simulink model "topic1——5"  (R2019b)
settings: Solver=VariableStepAuto  StartTime=0.0  StopTime=0.12  RelTol=1e-3
libraries: powerlib x14, powerlib_meascontrol x7
settings Model: Creator=96547  LastModifiedBy=96547

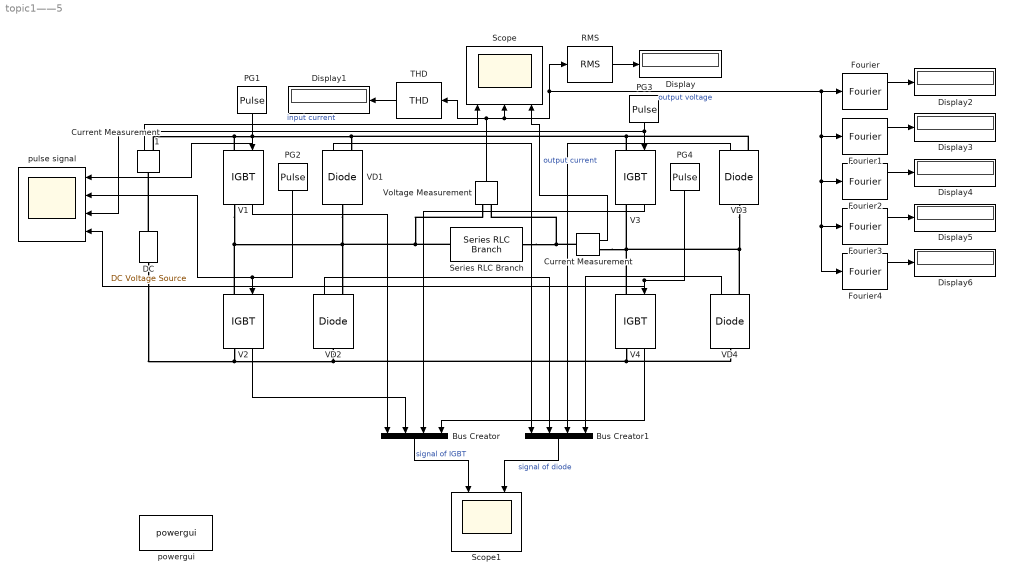
== system topic1——5 ==
  Bus Creator : BusCreator  Inputs=4
  Bus Creator1 : BusCreator  Inputs=4
  Current Measurement : powerlib/Measurements/Current Measurement  PhasorSimulation=off  OutputType=Complex  PSBequivalent=0
      settings: SourceProductName=Simscape Electrical
  Current Measurement1 : powerlib/Measurements/Current Measurement  PhasorSimulation=off  OutputType=Complex  PSBequivalent=0
      settings: SourceProductName=Simscape Electrical
  DC : powerlib/Electrical Sources/DC Voltage Source  Amplitude=400  Measurements=None
      settings: SourceProductName=Simscape Electrical
  Display{,1..6} (7 alike) : Display
  Fourier : powerlib_meascontrol/Measurements/Fourier  Freq=50  n=3  InInit=[0, 0]  Ts=0
      settings: SourceProductName=Simscape Electrical
  Fourier1 : powerlib_meascontrol/Measurements/Fourier  Freq=60  n=1  InInit=[0, 0]  Ts=0
      settings: SourceProductName=Simscape Electrical
  Fourier2 : powerlib_meascontrol/Measurements/Fourier  Freq=50  n=5  InInit=[0, 0]  Ts=0
      settings: SourceProductName=Simscape Electrical
  Fourier3 : powerlib_meascontrol/Measurements/Fourier  Freq=50  n=7  InInit=[0, 0]  Ts=0
      settings: SourceProductName=Simscape Electrical
  Fourier4 : powerlib_meascontrol/Measurements/Fourier  Freq=50  n=9  InInit=[0, 0]  Ts=0
      settings: SourceProductName=Simscape Electrical
  PG1 : DiscretePulseGenerator  PulseType=Time based  Period=0.02  PulseWidth=50
  PG2 : DiscretePulseGenerator  PulseType=Time based  Period=0.02  PulseWidth=50  PhaseDelay=0.01
  PG3 : DiscretePulseGenerator  PulseType=Time based  Period=0.02  PulseWidth=50  PhaseDelay=0.02*(1/6)
  PG4 : DiscretePulseGenerator  PulseType=Time based  Period=0.02  PulseWidth=50  PhaseDelay=0.01+0.02*(1/6)
  RMS : powerlib_meascontrol/Measurements/RMS  TrueRMS=on  Freq=60  RMSInit=120  Ts=0
      settings: SourceProductName=Simscape Electrical
  Scope : Scope  NumInputPorts=3
  Scope1 : Scope  NumInputPorts=2
  Series RLC Branch : powerlib/Elements/Series RLC Branch  LConnTagsString=__new0  RConnTagsString=__new0  BranchType=R  Resistance=8  Inductance=1e-3  SetiL0=off  InitialCurrent=0  Capacitance=1e-6  Setx0=off  InitialVoltage=0  Measurements=None
      settings: SourceProductName=Simscape Electrical
  THD : powerlib_meascontrol/Measurements/THD  Freq=60  Ts=0
      settings: SourceProductName=Simscape Electrical
  V{1..4} (4 alike) : powerlib/Power Electronics/IGBT  Ron=0.001  Lon=0  Vf=1  Tf=1e-6  Tt=2e-6  IC=0  Rs=1e5  Cs=inf  Measurements=on
      settings: SourceProductName=Simscape Electrical
  VD{1..4} (4 alike) : powerlib/Power Electronics/Diode  Ron=0.001  Lon=0  Vf=0.8  IC=0  UseSnubber=0  Rs=500  Cs=250e-9  Measurements=on
      settings: SourceProductName=Simscape Electrical
  Voltage Measurement : powerlib/Measurements/Voltage Measurement  PhasorSimulation=off  OutputType=Complex  PSBequivalent=0
      settings: SourceProductName=Simscape Electrical
  powergui : powerlib/powergui  Priority=1  SimulationMode=Continuous  SampleTime=50e-6  frequency=60  Iterations=50  frequencyindice=0  Pbase=100e6  ErrMax=1e-4  UnitsV=kV  UnitsW=MW  buscounter=0  FunctionMessages=off  echomessages=off  EnableUseOfTLC=off  CurrentSourceSwitches=off  DisableSnubberDevices=off  DisableRonSwitches=off  DisableVfSwitches=off  DisplayEquations=off  AutomaticDiscreteSolvers=off  SolverType=Tustin/Backward Euler (TBE)  Interpol=off  ExternalGateDelay=off  methode=off  Ts=100  x0status=blocks  SPID=on  SwTol=0  HookPort=off  NonlinearTolerance=1e-4  nMaxIteration=100  ContinueOnMaxIteration=off  RestoreLinks=warning  ResistiveCurrentMeasurement=off  Frange=[0:2:500]  Ylog=off  Xlog=on  ShowGrid=off  save=off  variable=ZData  structure=0  ZoomFFT=off  StartTime=0.0  cycles=1  DisplayStyle=1  fundamental=60  FreqAxis=off  MaxFrequency=1000  frequencyindicesteady=1  RmsSteady=1  display=off
      settings: SourceProductName=Simscape Electrical
  pulse signal : Scope  NumInputPorts=4
  wires:
  PG3/1 -> pulse signal/3, V3/1
  PG1/1 -> pulse signal/1, V1/1
  Voltage Measurement/1 -> Fourier1/1, Fourier2/1, Fourier3/1, Fourier4/1, Fourier/1, RMS/1, Scope/2, THD/1  "output voltage"
  Current Measurement/1 -> Scope/3  "output current"
  Bus Creator/1 -> Scope1/1  "signal of IGBT"
  V1/1 -> Bus Creator/1
  V2/1 -> Bus Creator/2
  V3/1 -> Bus Creator/3
  V4/1 -> Bus Creator/4
  VD4/1 -> Bus Creator1/4
  VD3/1 -> Bus Creator1/3
  VD1/1 -> Bus Creator1/1
  VD2/1 -> Bus Creator1/2
  Bus Creator1/1 -> Scope1/2  "signal of diode"
  RMS/1 -> Display/1
  THD/1 -> Display1/1
  Fourier/1 -> Display2/1
  Fourier1/1 -> Display3/1
  Fourier2/1 -> Display4/1
  Fourier3/1 -> Display5/1
  Fourier4/1 -> Display6/1
  PG2/1 -> pulse signal/2, V2/1
  PG4/1 -> pulse signal/4, V4/1
  Current Measurement1/1 -> Scope/1  "input current"
  connections:
  V1/LConn1 -- Current Measurement1/RConn1 -- VD3/RConn1 -- V3/LConn1 -- VD1/RConn1
  DC/LConn1 -- V2/RConn1 -- VD4/LConn1 -- V4/RConn1 -- VD2/LConn1
  VD1/LConn1 -- V2/LConn1 -- V1/RConn1 -- Voltage Measurement/LConn1 -- Series RLC Branch/RConn1 -- VD2/RConn1
  V4/LConn1 -- VD3/LConn1 -- VD4/RConn1 -- Current Measurement/RConn1 -- V3/RConn1
  Series RLC Branch/LConn1 -- Current Measurement/LConn1 -- Voltage Measurement/LConn2
  DC/RConn1 -- Current Measurement1/LConn1
